simulink model "StateWatcher_feedback"  (R2018b)
settings: Solver=VariableStepAuto  StartTime=0.0  StopTime=40  RelTol=1e-3  EnableMultiTasking=on
settings Model: Creator=B303  LastModifiedBy=erange
settings DataIOCC: LimitDataPoints=on
settings OptimizationCC: LifeSpan=inf
settings DebuggingCC: AllowSymbolicDim=off  SFUnexpectedBacktrackingDiag=warning  SFNoUnconditionalDefaultTransitionDiag=warning  SFExecutionAtInitializationDiag=none
settings ModelReferenceCC: PropagateSignalLabelsOutOfModel=off
settings SFSimCC: SimUseLocalCustomCode=off
settings RTWCC: RTWUseLocalCustomCode=off
settings CodeAppCC: StateflowObjectComments=on
settings GRTTargetCC: TargetLangStandard=C89/C90 (ANSI)
settings ConfigComp: CovMetricSettings=dw  CovHtmlReporting=on  CovSaveCumulativeToWorkspaceVar=on  CovSaveSingleToWorkspaceVar=on  CovExternalEMLEnable=off

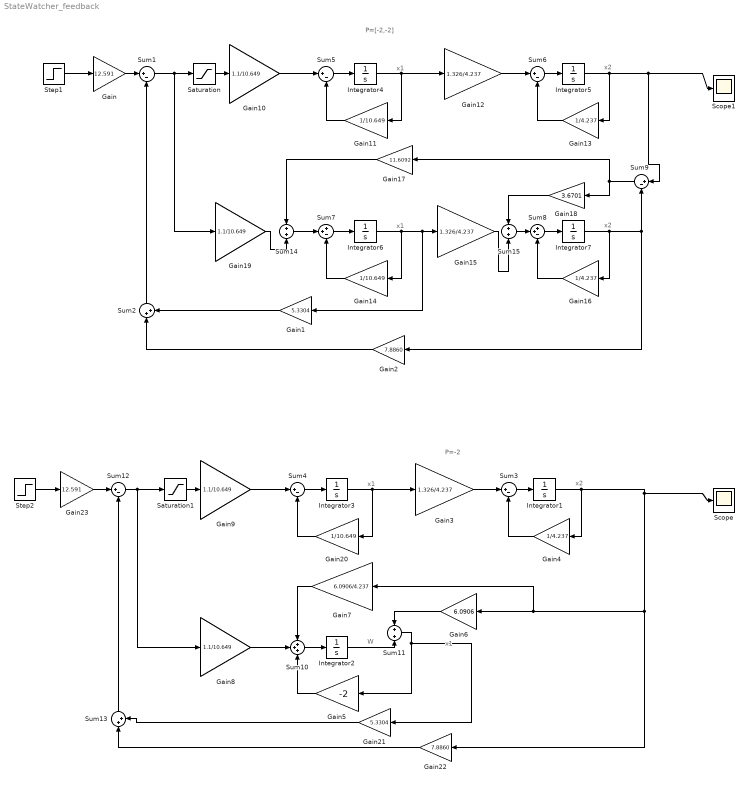
== system StateWatcher_feedback ==
  note: x2
  note: x2
  note: x1
  note: x1
  note: P=[-2,-2]
  note: x1
  note: P=-2
  note: x1
  note: W
  note: x2
  Gain : Gain  Gain=12.591
  Gain1 : Gain  Gain=5.3304
  Gain{8..10,19} (4 alike) : Gain  Gain=1.1/10.649
  Gain11 : Gain  Gain=1/10.649
  Gain12 : Gain  Gain=1.326/4.237
  Gain13 : Gain  Gain=1/4.237
  Gain14 : Gain  Gain=1/10.649
  Gain15 : Gain  Gain=1.326/4.237
  Gain16 : Gain  Gain=1/4.237
  Gain17 : Gain  Gain=11.6092
  Gain18 : Gain  Gain=3.6701
  Gain2 : Gain  Gain=7.8860
  Gain20 : Gain  Gain=1/10.649
  Gain21 : Gain  Gain=5.3304
  Gain22 : Gain  Gain=7.8860
  Gain23 : Gain  Gain=12.591
  Gain3 : Gain  Gain=1.326/4.237
  Gain4 : Gain  Gain=1/4.237
  Gain5 : Gain  Gain=-2
  Gain6 : Gain  Gain=6.0906
  Gain7 : Gain  Gain=6.0906/4.237
  Integrator{1..7} (7 alike) : Integrator
  Saturation : Saturate  UpperLimit=5  LowerLimit=0
  Saturation1 : Saturate  UpperLimit=5  LowerLimit=0
  Scope : Scope
  Scope1 : Scope
  Step1 : Step  Time=0  SampleTime=0
  Step2 : Step  Time=0  SampleTime=0
  Sum{1,3..6,9,12} (7 alike) : Sum  Inputs=|+-
  Sum10 : Sum  Inputs=+++
  Sum11 : Sum
  Sum13 : Sum  Inputs=|++
  Sum14 : Sum
  Sum15 : Sum
  Sum2 : Sum  Inputs=|++
  Sum7 : Sum  Inputs=++-
  Sum8 : Sum  Inputs=++-
  wires:
  Gain16/1 -> Sum8/3
  Gain14/1 -> Sum7/3
  Gain12/1 -> Sum6/1
  Step1/1 -> Gain/1
  Integrator5/1 -> Gain13/1, Sum9/1, Scope1/1
  Gain10/1 -> Sum5/1
  Gain13/1 -> Sum6/2
  Integrator4/1 -> Gain11/1, Gain12/1
  Sum5/1 -> Integrator4/1
  Sum7/1 -> Integrator6/1
  Integrator6/1 -> Gain14/1, Gain1/1, Gain15/1
  Sum8/1 -> Integrator7/1
  Sum6/1 -> Integrator5/1
  Integrator7/1 -> Sum9/2, Gain2/1, Gain16/1
  Gain11/1 -> Sum5/2
  Sum9/1 -> Gain17/1, Gain18/1
  Gain/1 -> Sum1/1
  Sum2/1 -> Sum1/2
  Gain1/1 -> Sum2/2
  Gain2/1 -> Sum2/1
  Sum1/1 -> Gain19/1, Saturation/1
  Saturation/1 -> Gain10/1
  Gain4/1 -> Sum3/2
  Gain8/1 -> Sum10/2
  Gain3/1 -> Sum3/1
  Integrator2/1 -> Sum11/2
  Integrator1/1 -> Gain4/1, Gain22/1, Gain7/1, Gain6/1, Scope/1
  Sum4/1 -> Integrator3/1
  Gain6/1 -> Sum11/1
  Sum3/1 -> Integrator1/1
  Gain5/1 -> Sum10/3
  Integrator3/1 -> Gain20/1, Gain3/1
  Sum10/1 -> Integrator2/1
  Gain20/1 -> Sum4/2
  Sum11/1 -> Gain5/1, Gain21/1
  Gain9/1 -> Sum4/1
  Gain7/1 -> Sum10/1
  Sum12/1 -> Gain8/1, Saturation1/1
  Gain23/1 -> Sum12/1
  Step2/1 -> Gain23/1
  Sum13/1 -> Sum12/2
  Gain22/1 -> Sum13/1
  Gain21/1 -> Sum13/2
  Sum14/1 -> Sum7/2
  Gain19/1 -> Sum14/2
  Gain17/1 -> Sum14/1
  Sum15/1 -> Sum8/2
  Gain15/1 -> Sum15/2
  Gain18/1 -> Sum15/1
  Saturation1/1 -> Gain9/1
